simulink model "Forward_control_Ref"  (R2013b)
settings: Solver=VariableStepDiscrete  StartTime=0.0  StopTime=inf  MaxStep=0.01  RelTol=1e-3
libraries: simulink x2
settings Model: Creator=Wasin  LastModifiedBy=Wasin

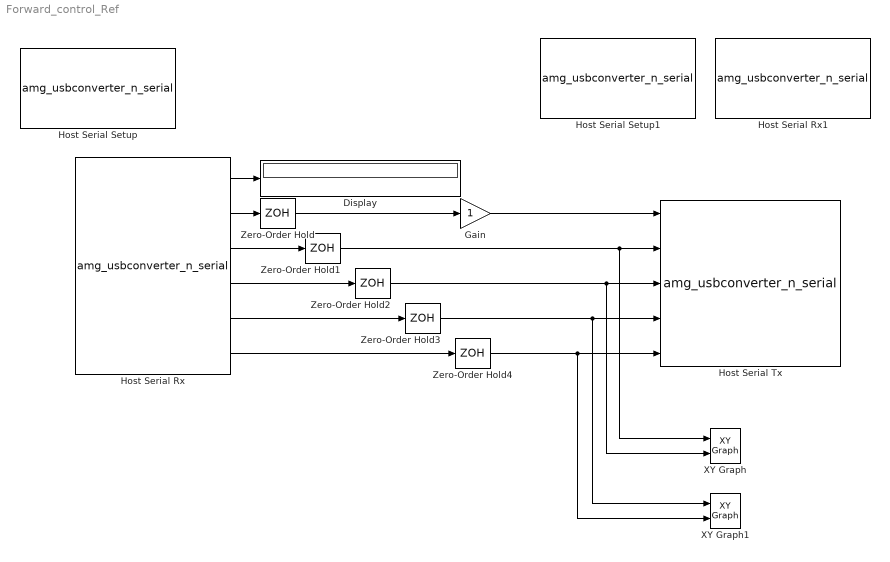
== system Forward_control_Ref ==
  Display : Display
  Gain : Gain  OutDataTypeStr=int8
  Host Serial Rx : S-Function  Priority=1  FunctionName=amg_usbconverter_n_serial  Parameters=configuration,port,transfer,baudrate,stopbit,inputtype,outputtype,binheaderarray,binterminatorarray,asciiheader,asciiterminator,bindatalength,packetmode,timeout,sampletime,initialvalues,blockid  EnableBusSupport=off  mask(amg_usbconverter_n_serial){configuration=Rx, port=COM22, baudrate=115200, databits=8, parity=None, stopbit=1, flowcontrol=None, advanceoptions=off, rxbuffersize=2048, txbuffersize=2048, transfer=Non-Blocking, enableinitial=off, initialvalues=[], timeout=20, packetmode=Binary, binheader='7E 7E', binterminator='03 03', porttype_double=0, porttype_single=0, porttype_int8=0, porttype_uint8=0, porttype_int16=5, porttype_uint16=0, porttype_int32=0, porttype_uint32=0, asciiformat='%d,%d,%d,%d,%d', rx_asciiterminator=LF (0x0A - "\n"), tx_asciiterminator=LF (0x0A - "\n"), inputtype=[0], outputtype=[6 3  4 4 4 4 4], binheaderarray=[2 126  126], binterminatorarray=[2 3  3], bindatalength=10, asciiheader=['%d,%d,%d,%d,%d' uint8(10)], asciiterminator=[1 10], sampletime=-1, sampletimestr=, blockid=HostSerialRx}
      mask prompts: baudrate "Baud rate (bps)"; databits "Data bits"; stopbit "Stop bit"; flowcontrol "Hardware flow control"; advanceoptions "Advance options"; rxbuffersize "Rx buffer size (bytes)"; txbuffersize "Tx buffer size (bytes)"; enableinitial "Enable initial value  (Closed loop HIL test)"; initialvalues "Initial values"; timeout "Wait time-out (Seconds)"; packetmode "Packet mode"; binheader "Binary header (example: '7E 7E')"; binterminator "Binary terminator (example: '03 03')"; porttype_double "Number of data port, type DOUBLE"; porttype_single "Number of data port, type SINGLE"; porttype_int8 "Number of data port, type INT8"; porttype_uint8 "Number of data port, type UINT8"; porttype_int16 "Number of data port, type INT16"; porttype_uint16 "Number of data port, type UINT16"; porttype_int32 "Number of data port, type INT32"; porttype_uint32 "Number of data port, type UINT32"; asciiformat "Ascii format"; rx_asciiterminator "End of packet"; tx_asciiterminator "End of packet"; inputtype "Input data type"; outputtype "Output data type"; binheaderarray "Binary header"; binterminatorarray "Binary terminator"; bindatalength "Binary data length"; asciiheader "Ascii header (printf format)"; asciiterminator "Ascii terminator"; sampletime "Sample time (sec)"; sampletimestr "Compiled sample time (sec) in string"
      mask help:
      | Enable initial value (Closed loop HIL test):
      |  - Checked: The block will return a initial value (constant) at first time step.
      |  - Unchecked: Normal operation, the block waiting for matched packet data before return value.
      mask init:
      | amg_usbconverter_n_serial_callback('init');
      mask Help: web(fullfile(waijungdocroot,'amg_usbconverter_n_uart.htm'), '-browser')
      mask TypeOptions configuration: Setup | Tx | Rx
      mask Callback configuration: amg_usbconverter_n_serial_callback('configuration');
      mask TypeOptions port: COM22
      mask Callback port: amg_usbconverter_n_serial_callback('port');
      mask Callback baudrate: amg_usbconverter_n_serial_callback('baudrate');
      mask TypeOptions databits: 8
      mask TypeOptions parity: None
      mask TypeOptions stopbit: 1 | 1.5 | 2
      mask TypeOptions flowcontrol: None | RTS | CTS | RTS/CTS
      mask Callback flowcontrol: amg_usbconverter_n_serial_callback('flowcontrol');
      mask Callback advanceoptions: amg_usbconverter_n_serial_callback('advanceoptions');
      mask TypeOptions rxbuffersize: 16 | 32 | 64 | 128 | 256 | 512 | 1024 | 2048
      mask TypeOptions txbuffersize: 16 | 32 | 64 | 128 | 256 | 512 | 1024 | 2048
      mask TypeOptions transfer: Blocking | Non-Blocking
      mask Callback transfer: amg_usbconverter_n_serial_callback('transfer');
      mask Callback enableinitial: amg_usbconverter_n_serial_callback('enableinitial');
      mask Callback initialvalues: amg_usbconverter_n_serial_callback('initialvalues');
      mask TypeOptions packetmode: Ascii | Binary
      mask Callback packetmode: amg_usbconverter_n_serial_callback('packetmode');
      mask Callback binheader: amg_usbconverter_n_serial_callback('binheader');
      mask Callback binterminator: amg_usbconverter_n_serial_callback('binterminator');
      mask Callback porttype_double: amg_usbconverter_n_serial_callback('porttype');
      mask Callback porttype_single: amg_usbconverter_n_serial_callback('porttype');
      mask Callback porttype_int8: amg_usbconverter_n_serial_callback('porttype');
      mask Callback porttype_uint8: amg_usbconverter_n_serial_callback('porttype');
      mask Callback porttype_int16: amg_usbconverter_n_serial_callback('porttype');
      mask Callback porttype_uint16: amg_usbconverter_n_serial_callback('porttype');
      mask Callback porttype_int32: amg_usbconverter_n_serial_callback('porttype');
      mask Callback porttype_uint32: amg_usbconverter_n_serial_callback('porttype');
      mask Callback asciiformat: amg_usbconverter_n_serial_callback('asciiformat');
      mask TypeOptions rx_asciiterminator: CR (0x0D - "\r") | LF (0x0A - "\n") | CRLF (0x0D 0x0A - "\r\n")
      mask Callback rx_asciiterminator: amg_usbconverter_n_serial_callback('rx_asciiterminator');
      mask TypeOptions tx_asciiterminator: CR (0x0D - "\r") | LF (0x0A - "\n") | CRLF (0x0D 0x0A - "\r\n") | None
      mask Callback tx_asciiterminator: amg_usbconverter_n_serial_callback('tx_asciiterminator');
      mask Callback sampletime: amg_usbconverter_n_serial_callback('sampletime');
      mask Callback sampletimestr: amg_usbconverter_n_serial_callback('sampletimestr');
      mask Callback blockid: amg_usbconverter_n_serial_callback('blockid');
      mask Display: text(0.05, 0.5, 'Port: COM22\nPacket: Binary\nTransfer: Non-Blocking\nTs (sec): 1','ver','middle','hor','left');port_label('output', 1,'READY');port_label('output', 2,'int16');port_label('output', 3,'int16');port_label('output', 4,'int16');port_label('output', 5,'int16');port_label('output', 6,'int16');
  Host Serial Rx1 : S-Function  Priority=1  FunctionName=amg_usbconverter_n_serial  Parameters=configuration,port,transfer,baudrate,stopbit,inputtype,outputtype,binheaderarray,binterminatorarray,asciiheader,asciiterminator,bindatalength,packetmode,timeout,sampletime,initialvalues,blockid  EnableBusSupport=off  mask(amg_usbconverter_n_serial){configuration=Rx, port=<Empty>, baudrate=115200, databits=8, parity=None, stopbit=1, flowcontrol=None, advanceoptions=off, rxbuffersize=2048, txbuffersize=2048, transfer=Blocking, enableinitial=off, initialvalues=[], timeout=20, packetmode=Binary, binheader='7E', binterminator='', porttype_double=0, porttype_single=0, porttype_int8=0, porttype_uint8=0, porttype_int16=0, porttype_uint16=0, porttype_int32=0, porttype_uint32=0, asciiformat='%d,%f', rx_asciiterminator=LF (0x0A - "\n"), tx_asciiterminator=LF (0x0A - "\n"), inputtype=[0], outputtype=[0 ], binheaderarray=[1 126], binterminatorarray=[0 ], bindatalength=0, asciiheader=['%d,%f' uint8(10)], asciiterminator=[1 10], sampletime=-1, sampletimestr=, blockid=HostSerialRx1}
      mask prompts: baudrate "Baud rate (bps)"; databits "Data bits"; stopbit "Stop bit"; flowcontrol "Hardware flow control"; advanceoptions "Advance options"; rxbuffersize "Rx buffer size (bytes)"; txbuffersize "Tx buffer size (bytes)"; enableinitial "Enable initial value  (Closed loop HIL test)"; initialvalues "Initial values"; timeout "Wait time-out (Seconds)"; packetmode "Packet mode"; binheader "Binary header (example: '7E 7E')"; binterminator "Binary terminator (example: '03 03')"; porttype_double "Number of data port, type DOUBLE"; porttype_single "Number of data port, type SINGLE"; porttype_int8 "Number of data port, type INT8"; porttype_uint8 "Number of data port, type UINT8"; porttype_int16 "Number of data port, type INT16"; porttype_uint16 "Number of data port, type UINT16"; porttype_int32 "Number of data port, type INT32"; porttype_uint32 "Number of data port, type UINT32"; asciiformat "Ascii format"; rx_asciiterminator "End of packet"; tx_asciiterminator "End of packet"; inputtype "Input data type"; outputtype "Output data type"; binheaderarray "Binary header"; binterminatorarray "Binary terminator"; bindatalength "Binary data length"; asciiheader "Ascii header (printf format)"; asciiterminator "Ascii terminator"; sampletime "Sample time (sec)"; sampletimestr "Compiled sample time (sec) in string"
      mask help:
      | Enable initial value (Closed loop HIL test):
      |  - Checked: The block will return a initial value (constant) at first time step.
      |  - Unchecked: Normal operation, the block waiting for matched packet data before return value.
      mask init:
      | amg_usbconverter_n_serial_callback('init');
      mask Help: web(fullfile(waijungdocroot,'amg_usbconverter_n_uart.htm'), '-browser')
      mask TypeOptions configuration: Setup | Tx | Rx
      mask Callback configuration: amg_usbconverter_n_serial_callback('configuration');
      mask TypeOptions port: <Empty>
      mask Callback port: amg_usbconverter_n_serial_callback('port');
      mask Callback baudrate: amg_usbconverter_n_serial_callback('baudrate');
      mask TypeOptions databits: 8
      mask TypeOptions parity: None
      mask TypeOptions stopbit: 1 | 1.5 | 2
      mask TypeOptions flowcontrol: None | RTS | CTS | RTS/CTS
      mask Callback flowcontrol: amg_usbconverter_n_serial_callback('flowcontrol');
      mask Callback advanceoptions: amg_usbconverter_n_serial_callback('advanceoptions');
      mask TypeOptions rxbuffersize: 16 | 32 | 64 | 128 | 256 | 512 | 1024 | 2048
      mask TypeOptions txbuffersize: 16 | 32 | 64 | 128 | 256 | 512 | 1024 | 2048
      mask TypeOptions transfer: Blocking | Non-Blocking
      mask Callback transfer: amg_usbconverter_n_serial_callback('transfer');
      mask Callback enableinitial: amg_usbconverter_n_serial_callback('enableinitial');
      mask Callback initialvalues: amg_usbconverter_n_serial_callback('initialvalues');
      mask TypeOptions packetmode: Ascii | Binary
      mask Callback packetmode: amg_usbconverter_n_serial_callback('packetmode');
      mask Callback binheader: amg_usbconverter_n_serial_callback('binheader');
      mask Callback binterminator: amg_usbconverter_n_serial_callback('binterminator');
      mask Callback porttype_double: amg_usbconverter_n_serial_callback('porttype');
      mask Callback porttype_single: amg_usbconverter_n_serial_callback('porttype');
      mask Callback porttype_int8: amg_usbconverter_n_serial_callback('porttype');
      mask Callback porttype_uint8: amg_usbconverter_n_serial_callback('porttype');
      mask Callback porttype_int16: amg_usbconverter_n_serial_callback('porttype');
      mask Callback porttype_uint16: amg_usbconverter_n_serial_callback('porttype');
      mask Callback porttype_int32: amg_usbconverter_n_serial_callback('porttype');
      mask Callback porttype_uint32: amg_usbconverter_n_serial_callback('porttype');
      mask Callback asciiformat: amg_usbconverter_n_serial_callback('asciiformat');
      mask TypeOptions rx_asciiterminator: CR (0x0D - "\r") | LF (0x0A - "\n") | CRLF (0x0D 0x0A - "\r\n")
      mask Callback rx_asciiterminator: amg_usbconverter_n_serial_callback('rx_asciiterminator');
      mask TypeOptions tx_asciiterminator: CR (0x0D - "\r") | LF (0x0A - "\n") | CRLF (0x0D 0x0A - "\r\n") | None
      mask Callback tx_asciiterminator: amg_usbconverter_n_serial_callback('tx_asciiterminator');
      mask Callback sampletime: amg_usbconverter_n_serial_callback('sampletime');
      mask Callback sampletimestr: amg_usbconverter_n_serial_callback('sampletimestr');
      mask Callback blockid: amg_usbconverter_n_serial_callback('blockid');
      mask Display: text(0.05, 0.5, 'Port: <Empty>\nPacket: Binary\nTransfer: Blocking\nTs (sec): 0','ver','middle','hor','left');
  Host Serial Setup : S-Function  Priority=1  FunctionName=amg_usbconverter_n_serial  Parameters=configuration,port,transfer,baudrate,stopbit,inputtype,outputtype,binheaderarray,binterminatorarray,asciiheader,asciiterminator,bindatalength,packetmode,timeout,sampletime,sampletimestr,blockid  EnableBusSupport=off  mask(amg_usbconverter_n_serial){configuration=Setup, port=COM22, baudrate=19200, databits=8, parity=None, stopbit=1, flowcontrol=None, advanceoptions=off, rxbuffersize=2048, txbuffersize=2048, transfer=Blocking, timeout=5, packetmode=Binary, binheader='7E 7E', binterminator='03 03', porttype_double=1, porttype_single=0, porttype_int8=1, porttype_uint8=0, porttype_int16=0, porttype_uint16=0, porttype_int32=0, porttype_uint32=0, asciiformat='%d,%f', rx_asciiterminator=CRLF (0x0D 0x0A - "\r\n"), tx_asciiterminator=CR (0x0D - "\r"), inputtype=[0], outputtype=[0], binheaderarray=[2 126  126], binterminatorarray=[2 3  3], bindatalength=0, asciiheader='', asciiterminator=[0], sampletime=inf, sampletimestr=, blockid=HostSerialSetup}
      mask prompts: baudrate "Baud rate (bps)"; databits "Data bits"; stopbit "Stop bit"; flowcontrol "Hardware flow control"; advanceoptions "Advance options"; rxbuffersize "Rx buffer size (bytes)"; txbuffersize "Tx buffer size (bytes)"; timeout "Wait time-out (Seconds)"; packetmode "Packet mode"; binheader "Binary header (example: '7E 7E')"; binterminator "Binary terminator (example: '03 03')"; porttype_double "Number of data port, type DOUBLE"; porttype_single "Number of data port, type SINGLE"; porttype_int8 "Number of data port, type INT8"; porttype_uint8 "Number of data port, type UINT8"; porttype_int16 "Number of data port, type INT16"; porttype_uint16 "Number of data port, type UINT16"; porttype_int32 "Number of data port, type INT32"; porttype_uint32 "Number of data port, type UINT32"; asciiformat "Ascii format"; rx_asciiterminator "End of packet"; tx_asciiterminator "End of packet"; inputtype "Input data type"; outputtype "Output data type"; binheaderarray "Binary header"; binterminatorarray "Binary terminator"; bindatalength "Binary data length"; asciiheader "Ascii header (printf format)"; asciiterminator "Ascii terminator"; sampletime "Sample time (sec)"; sampletimestr "Compiled sample time (sec) in string"
      mask init:
      | amg_usbconverter_n_serial_callback('init');
      mask Help: web(fullfile(waijungdocroot,'amg_usbconverter_n_uart.htm'), '-browser')
      mask TypeOptions configuration: Setup | Tx | Rx
      mask Callback configuration: amg_usbconverter_n_serial_callback('configuration');
      mask TypeOptions port: COM22
      mask Callback port: amg_usbconverter_n_serial_callback('port');
      mask Callback baudrate: amg_usbconverter_n_serial_callback('baudrate');
      mask TypeOptions databits: 8
      mask TypeOptions parity: None
      mask TypeOptions stopbit: 1 | 1.5 | 2
      mask TypeOptions flowcontrol: None | RTS | CTS | RTS/CTS
      mask Callback flowcontrol: amg_usbconverter_n_serial_callback('flowcontrol');
      mask Callback advanceoptions: amg_usbconverter_n_serial_callback('advanceoptions');
      mask TypeOptions rxbuffersize: 16 | 32 | 64 | 128 | 256 | 512 | 1024 | 2048
      mask TypeOptions txbuffersize: 16 | 32 | 64 | 128 | 256 | 512 | 1024 | 2048
      mask TypeOptions transfer: Blocking | Non-Blocking
      mask Callback transfer: amg_usbconverter_n_serial_callback('transfer');
      mask TypeOptions packetmode: Ascii | Binary
      mask Callback packetmode: amg_usbconverter_n_serial_callback('packetmode');
      mask Callback binheader: amg_usbconverter_n_serial_callback('binheader');
      mask Callback binterminator: amg_usbconverter_n_serial_callback('binterminator');
      mask Callback porttype_double: amg_usbconverter_n_serial_callback('porttype');
      mask Callback porttype_single: amg_usbconverter_n_serial_callback('porttype');
      mask Callback porttype_int8: amg_usbconverter_n_serial_callback('porttype');
      mask Callback porttype_uint8: amg_usbconverter_n_serial_callback('porttype');
      mask Callback porttype_int16: amg_usbconverter_n_serial_callback('porttype');
      mask Callback porttype_uint16: amg_usbconverter_n_serial_callback('porttype');
      mask Callback porttype_int32: amg_usbconverter_n_serial_callback('porttype');
      mask Callback porttype_uint32: amg_usbconverter_n_serial_callback('porttype');
      mask Callback asciiformat: amg_usbconverter_n_serial_callback('asciiformat');
      mask TypeOptions rx_asciiterminator: CR (0x0D - "\r") | LF (0x0A - "\n") | CRLF (0x0D 0x0A - "\r\n")
      mask Callback rx_asciiterminator: amg_usbconverter_n_serial_callback('rx_asciiterminator');
      mask TypeOptions tx_asciiterminator: CR (0x0D - "\r") | LF (0x0A - "\n") | CRLF (0x0D 0x0A - "\r\n") | None
      mask Callback tx_asciiterminator: amg_usbconverter_n_serial_callback('tx_asciiterminator');
      mask Callback sampletime: amg_usbconverter_n_serial_callback('sampletime');
      mask Callback sampletimestr: amg_usbconverter_n_serial_callback('sampletimestr');
      mask Callback blockid: amg_usbconverter_n_serial_callback('blockid');
      mask Display: text(0.5, 0.5, 'Port: COM22\nBaud (Bps): 19200\nFrame: 8-None-1','ver','middle','hor','center');
  Host Serial Setup1 : S-Function  Priority=1  FunctionName=amg_usbconverter_n_serial  Parameters=configuration,port,transfer,baudrate,stopbit,inputtype,outputtype,binheaderarray,binterminatorarray,asciiheader,asciiterminator,bindatalength,packetmode,timeout,sampletime,sampletimestr,blockid  EnableBusSupport=off  mask(amg_usbconverter_n_serial){configuration=Setup, port=<Empty>, baudrate=115200, databits=8, parity=None, stopbit=1, flowcontrol=None, advanceoptions=off, rxbuffersize=2048, txbuffersize=2048, transfer=Blocking, timeout=5, packetmode=Binary, binheader='7E 7E', binterminator='03 03', porttype_double=1, porttype_single=0, porttype_int8=1, porttype_uint8=0, porttype_int16=0, porttype_uint16=0, porttype_int32=0, porttype_uint32=0, asciiformat='%d,%f', rx_asciiterminator=CRLF (0x0D 0x0A - "\r\n"), tx_asciiterminator=CR (0x0D - "\r"), inputtype=[0], outputtype=[0], binheaderarray=[2 126  126], binterminatorarray=[2 3  3], bindatalength=0, asciiheader='', asciiterminator=[0], sampletime=inf, sampletimestr=, blockid=HostSerialSetup}
      mask prompts: baudrate "Baud rate (bps)"; databits "Data bits"; stopbit "Stop bit"; flowcontrol "Hardware flow control"; advanceoptions "Advance options"; rxbuffersize "Rx buffer size (bytes)"; txbuffersize "Tx buffer size (bytes)"; timeout "Wait time-out (Seconds)"; packetmode "Packet mode"; binheader "Binary header (example: '7E 7E')"; binterminator "Binary terminator (example: '03 03')"; porttype_double "Number of data port, type DOUBLE"; porttype_single "Number of data port, type SINGLE"; porttype_int8 "Number of data port, type INT8"; porttype_uint8 "Number of data port, type UINT8"; porttype_int16 "Number of data port, type INT16"; porttype_uint16 "Number of data port, type UINT16"; porttype_int32 "Number of data port, type INT32"; porttype_uint32 "Number of data port, type UINT32"; asciiformat "Ascii format"; rx_asciiterminator "End of packet"; tx_asciiterminator "End of packet"; inputtype "Input data type"; outputtype "Output data type"; binheaderarray "Binary header"; binterminatorarray "Binary terminator"; bindatalength "Binary data length"; asciiheader "Ascii header (printf format)"; asciiterminator "Ascii terminator"; sampletime "Sample time (sec)"; sampletimestr "Compiled sample time (sec) in string"
      mask init:
      | amg_usbconverter_n_serial_callback('init');
      mask Help: web(fullfile(waijungdocroot,'amg_usbconverter_n_uart.htm'), '-browser')
      mask TypeOptions configuration: Setup | Tx | Rx
      mask Callback configuration: amg_usbconverter_n_serial_callback('configuration');
      mask TypeOptions port: COM22 | <Empty>
      mask Callback port: amg_usbconverter_n_serial_callback('port');
      mask Callback baudrate: amg_usbconverter_n_serial_callback('baudrate');
      mask TypeOptions databits: 8
      mask TypeOptions parity: None
      mask TypeOptions stopbit: 1 | 1.5 | 2
      mask TypeOptions flowcontrol: None | RTS | CTS | RTS/CTS
      mask Callback flowcontrol: amg_usbconverter_n_serial_callback('flowcontrol');
      mask Callback advanceoptions: amg_usbconverter_n_serial_callback('advanceoptions');
      mask TypeOptions rxbuffersize: 16 | 32 | 64 | 128 | 256 | 512 | 1024 | 2048
      mask TypeOptions txbuffersize: 16 | 32 | 64 | 128 | 256 | 512 | 1024 | 2048
      mask TypeOptions transfer: Blocking | Non-Blocking
      mask Callback transfer: amg_usbconverter_n_serial_callback('transfer');
      mask TypeOptions packetmode: Ascii | Binary
      mask Callback packetmode: amg_usbconverter_n_serial_callback('packetmode');
      mask Callback binheader: amg_usbconverter_n_serial_callback('binheader');
      mask Callback binterminator: amg_usbconverter_n_serial_callback('binterminator');
      mask Callback porttype_double: amg_usbconverter_n_serial_callback('porttype');
      mask Callback porttype_single: amg_usbconverter_n_serial_callback('porttype');
      mask Callback porttype_int8: amg_usbconverter_n_serial_callback('porttype');
      mask Callback porttype_uint8: amg_usbconverter_n_serial_callback('porttype');
      mask Callback porttype_int16: amg_usbconverter_n_serial_callback('porttype');
      mask Callback porttype_uint16: amg_usbconverter_n_serial_callback('porttype');
      mask Callback porttype_int32: amg_usbconverter_n_serial_callback('porttype');
      mask Callback porttype_uint32: amg_usbconverter_n_serial_callback('porttype');
      mask Callback asciiformat: amg_usbconverter_n_serial_callback('asciiformat');
      mask TypeOptions rx_asciiterminator: CR (0x0D - "\r") | LF (0x0A - "\n") | CRLF (0x0D 0x0A - "\r\n")
      mask Callback rx_asciiterminator: amg_usbconverter_n_serial_callback('rx_asciiterminator');
      mask TypeOptions tx_asciiterminator: CR (0x0D - "\r") | LF (0x0A - "\n") | CRLF (0x0D 0x0A - "\r\n") | None
      mask Callback tx_asciiterminator: amg_usbconverter_n_serial_callback('tx_asciiterminator');
      mask Callback sampletime: amg_usbconverter_n_serial_callback('sampletime');
      mask Callback sampletimestr: amg_usbconverter_n_serial_callback('sampletimestr');
      mask Callback blockid: amg_usbconverter_n_serial_callback('blockid');
      mask Display: text(0.5, 0.5, 'Port: <Empty>\nBaud (Bps): 115200\nFrame: 8-None-1','ver','middle','hor','center');
  Host Serial Tx : S-Function  Priority=1  FunctionName=amg_usbconverter_n_serial  Parameters=configuration,port,transfer,baudrate,stopbit,inputtype,outputtype,binheaderarray,binterminatorarray,asciiheader,asciiterminator,bindatalength,packetmode,timeout,sampletime,sampletimestr,blockid  EnableBusSupport=off  mask(amg_usbconverter_n_serial){configuration=Tx, port=<Empty>, baudrate=115200, databits=8, parity=None, stopbit=1, flowcontrol=None, advanceoptions=off, rxbuffersize=2048, txbuffersize=2048, transfer=Blocking, timeout=20, packetmode=Binary, binheader='', binterminator='', porttype_double=0, porttype_single=0, porttype_int8=1, porttype_uint8=0, porttype_int16=4, porttype_uint16=0, porttype_int32=0, porttype_uint32=0, asciiformat='%d,%f', rx_asciiterminator=CRLF (0x0D 0x0A - "\r\n"), tx_asciiterminator=LF (0x0A - "\n"), inputtype=[5  2 4 4 4 4], outputtype=[0], binheaderarray=[0 ], binterminatorarray=[0 ], bindatalength=9, asciiheader=['%d,%f' uint8(10)], asciiterminator=[1 10], sampletime=-1, sampletimestr=, blockid=HostSerialTx}
      mask prompts: baudrate "Baud rate (bps)"; databits "Data bits"; stopbit "Stop bit"; flowcontrol "Hardware flow control"; advanceoptions "Advance options"; rxbuffersize "Rx buffer size (bytes)"; txbuffersize "Tx buffer size (bytes)"; timeout "Wait time-out (Seconds)"; packetmode "Packet mode"; binheader "Binary header (example: '7E 7E')"; binterminator "Binary terminator (example: '03 03')"; porttype_double "Number of data port, type DOUBLE"; porttype_single "Number of data port, type SINGLE"; porttype_int8 "Number of data port, type INT8"; porttype_uint8 "Number of data port, type UINT8"; porttype_int16 "Number of data port, type INT16"; porttype_uint16 "Number of data port, type UINT16"; porttype_int32 "Number of data port, type INT32"; porttype_uint32 "Number of data port, type UINT32"; asciiformat "Ascii format"; rx_asciiterminator "End of packet"; tx_asciiterminator "End of packet"; inputtype "Input data type"; outputtype "Output data type"; binheaderarray "Binary header"; binterminatorarray "Binary terminator"; bindatalength "Binary data length"; asciiheader "Ascii header (printf format)"; asciiterminator "Ascii terminator"; sampletime "Sample time (sec)"; sampletimestr "Compiled sample time (sec) in string"
      mask init:
      | amg_usbconverter_n_serial_callback('init');
      mask Help: web(fullfile(waijungdocroot,'amg_usbconverter_n_uart.htm'), '-browser')
      mask TypeOptions configuration: Setup | Tx | Rx
      mask Callback configuration: amg_usbconverter_n_serial_callback('configuration');
      mask TypeOptions port: <Empty>
      mask Callback port: amg_usbconverter_n_serial_callback('port');
      mask Callback baudrate: amg_usbconverter_n_serial_callback('baudrate');
      mask TypeOptions databits: 8
      mask TypeOptions parity: None
      mask TypeOptions stopbit: 1 | 1.5 | 2
      mask TypeOptions flowcontrol: None | RTS | CTS | RTS/CTS
      mask Callback flowcontrol: amg_usbconverter_n_serial_callback('flowcontrol');
      mask Callback advanceoptions: amg_usbconverter_n_serial_callback('advanceoptions');
      mask TypeOptions rxbuffersize: 16 | 32 | 64 | 128 | 256 | 512 | 1024 | 2048
      mask TypeOptions txbuffersize: 16 | 32 | 64 | 128 | 256 | 512 | 1024 | 2048
      mask TypeOptions transfer: Blocking | Non-Blocking
      mask Callback transfer: amg_usbconverter_n_serial_callback('transfer');
      mask TypeOptions packetmode: Ascii | Binary
      mask Callback packetmode: amg_usbconverter_n_serial_callback('packetmode');
      mask Callback binheader: amg_usbconverter_n_serial_callback('binheader');
      mask Callback binterminator: amg_usbconverter_n_serial_callback('binterminator');
      mask Callback porttype_double: amg_usbconverter_n_serial_callback('porttype');
      mask Callback porttype_single: amg_usbconverter_n_serial_callback('porttype');
      mask Callback porttype_int8: amg_usbconverter_n_serial_callback('porttype');
      mask Callback porttype_uint8: amg_usbconverter_n_serial_callback('porttype');
      mask Callback porttype_int16: amg_usbconverter_n_serial_callback('porttype');
      mask Callback porttype_uint16: amg_usbconverter_n_serial_callback('porttype');
      mask Callback porttype_int32: amg_usbconverter_n_serial_callback('porttype');
      mask Callback porttype_uint32: amg_usbconverter_n_serial_callback('porttype');
      mask Callback asciiformat: amg_usbconverter_n_serial_callback('asciiformat');
      mask TypeOptions rx_asciiterminator: CR (0x0D - "\r") | LF (0x0A - "\n") | CRLF (0x0D 0x0A - "\r\n")
      mask Callback rx_asciiterminator: amg_usbconverter_n_serial_callback('rx_asciiterminator');
      mask TypeOptions tx_asciiterminator: CR (0x0D - "\r") | LF (0x0A - "\n") | CRLF (0x0D 0x0A - "\r\n") | None
      mask Callback tx_asciiterminator: amg_usbconverter_n_serial_callback('tx_asciiterminator');
      mask Callback sampletime: amg_usbconverter_n_serial_callback('sampletime');
      mask Callback sampletimestr: amg_usbconverter_n_serial_callback('sampletimestr');
      mask Callback blockid: amg_usbconverter_n_serial_callback('blockid');
      mask Display: text(0.95, 0.5, 'Port: <Empty>\nPacket: Binary\nTransfer: Blocking\nTs (sec): 0','ver','middle','hor','right');port_label('input', 1,'int8');port_label('input', 2,'int16');port_label('input', 3,'int16');port_label('input', 4,'int16');port_label('input', 5,'int16');
  XY Graph : simulink/Sinks/XY Graph  xmin=-100  xmax=100  ymin=-100  ymax=100  st=-1
  XY Graph1 : simulink/Sinks/XY Graph  xmin=-100  xmax=100  ymin=-100  ymax=100  st=-1
  Zero-Order Hold{,1..4} (5 alike) : ZeroOrderHold
  wires:
  Host Serial Rx/1 -> Display/1
  Host Serial Rx/2 -> Zero-Order Hold/1
  Host Serial Rx/3 -> Zero-Order Hold1/1
  Host Serial Rx/4 -> Zero-Order Hold2/1
  Host Serial Rx/5 -> Zero-Order Hold3/1
  Host Serial Rx/6 -> Zero-Order Hold4/1
  Zero-Order Hold/1 -> Gain/1
  Zero-Order Hold1/1 -> Host Serial Tx/2, XY Graph/1
  Zero-Order Hold2/1 -> Host Serial Tx/3, XY Graph/2
  Zero-Order Hold3/1 -> Host Serial Tx/4, XY Graph1/1
  Zero-Order Hold4/1 -> Host Serial Tx/5, XY Graph1/2
  Gain/1 -> Host Serial Tx/1
